simulink model "HighOrderModulatorPSK8"  (R2020a)
settings: Solver=VariableStepAuto  StartTime=0.0  StopTime=10  RelTol=1e-3
libraries: commdigbbndpm3 x2, commchan3 x1, commrandsrc3 x1, commsink2 x1
settings Model: Creator=se305  LastModifiedBy=sergioe
settings SFSimCC: CustomCodeUndefinedFunction=UseInterfaceOnly

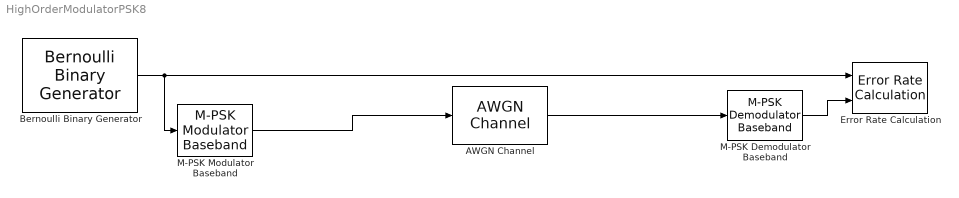
== system HighOrderModulatorPSK8 ==
  AWGN Channel : commchan3/AWGN Channel  InputProcessing=Columns as channels (frame based)  seed=67  noiseMode="Signal to noise ratio  (Eb/No)"  EbNodB=EbNo  EsNodB=10  SNRdB=10  bitsPerSym=3  Ps=1/4  Tsym=0.003  variance=1
  Bernoulli Binary Generator : commrandsrc3/Bernoulli Binary Generator  ProbabilityOfZero=0.5  SeedSource=Auto  Seed=0  SampleTime=0.001  SamplesPerFrame=3  OutputDataType=double  SimulateUsing=Interpreted execution
  Error Rate Calculation : commsink2/Error Rate Calculation  N=0  st_delay=0  cp_mode=Entire frame  subframe=[]  PMode=Workspace  WsName=ErrorVec  RsMode2=off  stop=off  numErr=100  maxBits=1e6
  M-PSK Demodulator Baseband : commdigbbndpm3/M-PSK Demodulator Baseband  M=8  OutType=Integer  DecType=Hard decision  VarSource=Dialog  Variance=1  Dec=Binary  Mapping=[0:7]  Ph=0  outDtype1=Inherit via internal rule  outDtype2=Inherit via internal rule  derotateFactorWordLen=16  derotateFactorDataTypeStr=Inherit: Same word length as input  derotateFactorLastDataTypeStr=Inherit: Same word length as input
  M-PSK Modulator Baseband : commdigbbndpm3/M-PSK Modulator Baseband  M=8  InType=Integer  Enc=Binary  Mapping=[0:7]  Ph=0  outDtype=double  outWordLen=16  outUDDataType=sfix(16)  outFracLenMode=Best precision  outFracLen=15  outDataTypeStr=double  outLastDataTypeStr=double
  wires:
  Bernoulli Binary Generator/1 -> M-PSK Modulator Baseband/1, Error Rate Calculation/1
  M-PSK Modulator Baseband/1 -> AWGN Channel/1
  AWGN Channel/1 -> M-PSK Demodulator Baseband/1
  M-PSK Demodulator Baseband/1 -> Error Rate Calculation/2
